simulink library "pmm"  (R2021b)
settings: Solver=VariableStepAuto  StartTime=0.0  StopTime=10.0  RelTol=1e-3
undefined symbols (not defined in the file or in its folder): APMM_CoolgFanActCurr_X_pct, APMM_EWP1Curr_X_c, APMM_EWP3Curr_X_c, APMM_LVBattChktime_X_enum, APMM_LVBattChrgtime_X_enum, APMM_LVChrgLv_X_mV, ENUM_ANTITHEFT_ALARM, ENUM_ANTITHEFT_ARM, ENUM_ANTITHEFT_DISARM, ENUM_ANTITHEFT_WAIT, ENUM_CHRGPLUGSTA_NONE, ENUM_CRASHSTATE_NOCRASH, ENUM_DCDCFAULTSTA_ANYFAULTLV1, ENUM_DCDCFAULTSTA_ANYFAULTLV2, ENUM_DRIVETRAIN_AWD, ENUM_DRIVETRAIN_FWD, ENUM_DRIVETRAIN_RWD, ENUM_GEARACTUALPOSN_D, ENUM_GEARACTUALPOSN_N, ENUM_GEARACTUALPOSN_R, ENUM_HVBATTREADYPRE_READY, ENUM_OTACHKSTA_NOREQUEST, ENUM_OTACHKSTA_NOTIMEOUT, ENUM_OTACHKSTA_TIMEOUT, ENUM_PDKEYRAWLULOCK_INLOCK, ENUM_PDKEYRAWLULOCK_INUNLOCK, ENUM_PDKEYRAWPS_INPS, ENUM_PDKEYSTA_LOCK, ENUM_PDKEYSTA_PS, ENUM_PDKEYSTA_UNAVALIABLE, ENUM_PDKEYSTA_UNLOCK, ENUM_POWERSTA_OFF, ENUM_POWERSTA_OFFC, ENUM_POWERSTA_STANDBY, ENUM_PWRREQOTA_REQPOWEROFF, ENUM_PWRREQOTA_REQPOWERSTDBY, ENUM_PWRSTASW_READY, FALSE, KPMM_AllDoorClosedHoldTime_s, KPMM_APSAllowThd_pct, KPMM_BattDownFailtime_s, KPMM_BattUpFailtime_s, KPMM_BattUpResetRty_cnt, KPMM_BattUpResetSW_flg, KPMM_BattUpResetTO_s, KPMM_BattUpRstDlyTO_s, KPMM_BrakeSWHoldTime_s, KPMM_ChrgPlugHoldTime_s, KPMM_DCDCDisableFailtime_s, KPMM_DCDCEnableFailtime_s, KPMM_DCDCVSET_V, KPMM_DCDCVSETLVChrg_V, KPMM_DoorSWHoldTime_s, KPMM_DriverSafetyChkFailtime_s, KPMM_DrivetrainSelect_enum_ovrdflg, KPMM_DrivetrainSelect_enum_ovrdval, KPMM_FDADC12VDetAccu_s, KPMM_FDADC12VDetAccuIntval_s, KPMM_FirstLVCheckHoldT_s, KPMM_FrMCUDischrgVolt_V ... (+54)
libraries: simulink x28, hcu_lib x13
(part 3 of 5)

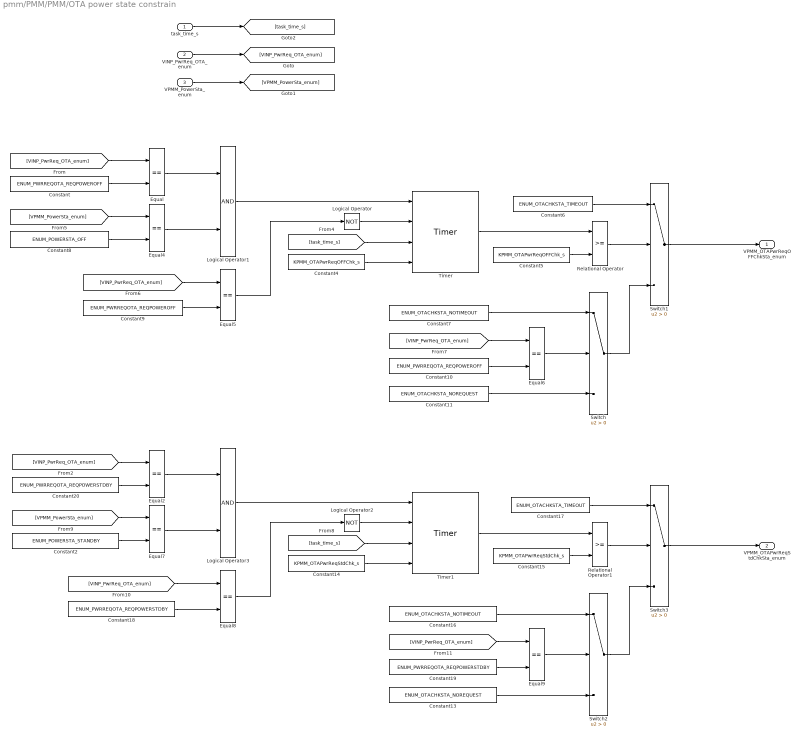
== system pmm/PMM/PMM/OTA power state constrain ==
  task_time_s : Inport
  VINP_PwrReq_OTA_enum : Inport  Port=2
  VPMM_PowerSta_enum : Inport  Port=3
  Constant : Constant  Value=ENUM_PWRREQOTA_REQPOWEROFF
  Constant10 : Constant  Value=ENUM_PWRREQOTA_REQPOWEROFF
  Constant11 : Constant  Value=ENUM_OTACHKSTA_NOREQUEST
  Constant13 : Constant  Value=ENUM_OTACHKSTA_NOREQUEST
  Constant14 : Constant  Value=KPMM_OTAPwrReqStdChk_s
  Constant15 : Constant  Value=KPMM_OTAPwrReqStdChk_s
  Constant16 : Constant  Value=ENUM_OTACHKSTA_NOTIMEOUT
  Constant17 : Constant  Value=ENUM_OTACHKSTA_TIMEOUT
  Constant18 : Constant  Value=ENUM_PWRREQOTA_REQPOWERSTDBY
  Constant19 : Constant  Value=ENUM_PWRREQOTA_REQPOWERSTDBY
  Constant2 : Constant  Value=ENUM_POWERSTA_STANDBY
  Constant20 : Constant  Value=ENUM_PWRREQOTA_REQPOWERSTDBY
  Constant4 : Constant  Value=KPMM_OTAPwrReqOFFChk_s
  Constant5 : Constant  Value=KPMM_OTAPwrReqOFFChk_s
  Constant6 : Constant  Value=ENUM_OTACHKSTA_TIMEOUT
  Constant7 : Constant  Value=ENUM_OTACHKSTA_NOTIMEOUT
  Constant8 : Constant  Value=ENUM_POWERSTA_OFF
  Constant9 : Constant  Value=ENUM_PWRREQOTA_REQPOWEROFF
  Equal{,2,4..9} (8 alike) : RelationalOperator  Operator===  OutDataTypeStr=boolean  RndMeth=Simplest
  Logical Operator : Logic  Operator=NOT  AllPortsSameDT=off  OutDataTypeStr=boolean
  Logical Operator1 : Logic  AllPortsSameDT=off  OutDataTypeStr=boolean
  Logical Operator2 : Logic  Operator=NOT  AllPortsSameDT=off  OutDataTypeStr=boolean
  Logical Operator3 : Logic  AllPortsSameDT=off  OutDataTypeStr=boolean
  Relational Operator : RelationalOperator  OutDataTypeStr=boolean  RndMeth=Simplest
  Relational Operator1 : RelationalOperator  OutDataTypeStr=boolean  RndMeth=Simplest
  Switch{,1..3} (4 alike) : Switch  Criteria=u2 > Threshold
  Timer : hcu_lib/Basic_Blocks/Timer
  Timer1 : hcu_lib/Basic_Blocks/Timer
  VPMM_OTAPwrReqOFFChkSta_enum : Outport
  VPMM_OTAPwrReqStdChkSta_enum : Outport  Port=2
  wires:
  Constant/1 -> Equal/2
  VINP_PwrReq_OTA_enum/1 -> [VINP_PwrReq_OTA_enum]
  VPMM_PowerSta_enum/1 -> [VPMM_PowerSta_enum]
  [VINP_PwrReq_OTA_enum] -> Equal/1
  task_time_s/1 -> [task_time_s]
  [task_time_s] -> Timer/3
  Constant4/1 -> Timer/4
  Constant5/1 -> Relational Operator/2
  Timer/1 -> Relational Operator/1
  Relational Operator/1 -> Switch1/2
  Logical Operator/1 -> Timer/2
  Constant8/1 -> Equal4/2
  [VPMM_PowerSta_enum] -> Equal4/1
  Equal/1 -> Logical Operator1/1
  Equal4/1 -> Logical Operator1/2
  Logical Operator1/1 -> Timer/1
  [VINP_PwrReq_OTA_enum] -> Equal5/1
  Constant9/1 -> Equal5/2
  Equal5/1 -> Logical Operator/1
  Constant6/1 -> Switch1/1
  Constant10/1 -> Equal6/2
  [VINP_PwrReq_OTA_enum] -> Equal6/1
  Equal6/1 -> Switch/2
  Constant7/1 -> Switch/1
  Switch/1 -> Switch1/3
  Constant11/1 -> Switch/3
  Switch1/1 -> VPMM_OTAPwrReqOFFChkSta_enum/1
  Switch2/1 -> Switch3/3
  Equal9/1 -> Switch2/2
  [VINP_PwrReq_OTA_enum] -> Equal9/1
  Equal8/1 -> Logical Operator2/1
  [VINP_PwrReq_OTA_enum] -> Equal8/1
  Logical Operator3/1 -> Timer1/1
  Equal7/1 -> Logical Operator3/2
  Equal2/1 -> Logical Operator3/1
  [VPMM_PowerSta_enum] -> Equal7/1
  Logical Operator2/1 -> Timer1/2
  Relational Operator1/1 -> Switch3/2
  Timer1/1 -> Relational Operator1/1
  Constant15/1 -> Relational Operator1/2
  Constant14/1 -> Timer1/4
  [task_time_s] -> Timer1/3
  [VINP_PwrReq_OTA_enum] -> Equal2/1
  Constant20/1 -> Equal2/2
  Constant13/1 -> Switch2/3
  Constant16/1 -> Switch2/1
  Constant17/1 -> Switch3/1
  Switch3/1 -> VPMM_OTAPwrReqStdChkSta_enum/1
  Constant2/1 -> Equal7/2
  Constant18/1 -> Equal8/2
  Constant19/1 -> Equal9/2

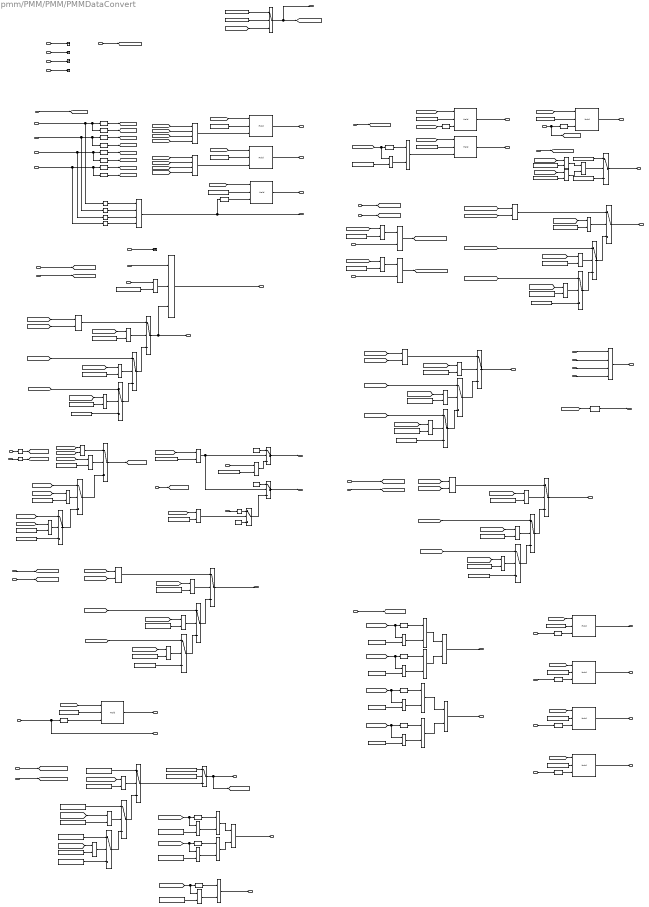
== system pmm/PMM/PMM/PMMDataConvert ==
  note: Detect HV power state
  note: Detect PW Continue Use
  note: Detect SchedChgwake
  note: Detect IVI Power OFF
  note: Monitor for DCDC fault level
  note: VPMM_SafetyChkMLv_flg
      | 0 Fail
      | 1 OK
  note: Safety Check
  note: VPMM_TMSpdThdSta_flg
      | 0 = Not allow MCU disable
      | 1 = Allow MCU disable
  note: 0 = HVIL close; 1 = HVIL open
  note: Seat Switch Rising Edge
  note: Detect Gun Plug Rising/Faling Edge
  note: KEY STATE
  note: Brake signal convert to rising edge
  note: Door judgement
  note: Precharge Check
  note: MCU Enable
  note: MCU Discharge
  note: MCU Ready
  note: Antitheft State
  note: OPDS Signal tramsmit function
  note: BMSWarn judgement
  note: MCU DC Bus Max Voltage judgement
  task_time_s : Inport
  VBCM_AntitheftSta_enum : Inport  Port=2
  VINP_DrDoorSW_flg : Inport  Port=3
  VINP_PsDoorSW_flg : Inport  Port=4
  VINP_RRDoorSW_flg : Inport  Port=5
  VINP_RLDoorSW_flg : Inport  Port=6
  VINP_BrakeSWGPIO_flg : Inport  Port=7
  VINP_FrMCUDCBusVolt_V : Inport  Port=8
  VINP_FrMCUDischrgSta_flg : Inport  Port=9
  VINP_FrMCUEnaSta_flg : Inport  Port=10
  VINP_FrMCUErr_enum : Inport  Port=11
  VINP_FrMCUReady4Pre_flg : Inport  Port=12
  VINP_FrMCUReady_flg : Inport  Port=13
  VINP_FrMCUTemp_C : Inport  Port=14
  VINP_RrMCUDCBusVolt_V : Inport  Port=15
  VINP_RrMCUDischrgSta_flg : Inport  Port=16
  VINP_RrMCUEnaSta_flg : Inport  Port=17
  VINP_RrMCUErr_enum : Inport  Port=18
  VINP_RrMCUReady4Pre_flg : Inport  Port=19
  VINP_RrMCUReady_flg : Inport  Port=20
  VINP_RrMCUTemp_C : Inport  Port=21
  VINP_DCDCReady4Pre_flg : Inport  Port=22
  VINP_OBCReady4Pre_flg : Inport  Port=23
  VINP_HVBattReady4Pre_enum : Inport  Port=24
  VINP_PDKeyAreaPS_enum : Inport  Port=25
  VINP_PDKeyAreaLockUnlock_enum : Inport  Port=26
  VINP_ChrgPlugSta_enum : Inport  Port=27
  VINP_SeatSW_flg : Inport  Port=28
  VINP_HVILSta_flg : Inport  Port=29
  VINP_CrashOutputSts_enum : Inport  Port=30
  VPMM_PowerSta_enum : Inport  Port=31
  VINP_RrTMSpd_rpm : Inport  Port=32
  VINP_FrTMSpd_rpm : Inport  Port=33
  VINP_BMSWarn5_flg : Inport  Port=34
  VINP_BMSWarn6_flg : Inport  Port=35
  VINP_BMSWarn7_flg : Inport  Port=36
  VINP_BMSWarn8_flg : Inport  Port=37
  VINP_DrivetrainSelect_enum : Inport  Port=38
  VINP_DCDCFaultSta_enum : Inport  Port=39
  VINP_IVIPwroffreq_flg : Inport  Port=40
  VINP_SchedChgwake_flg : Inport  Port=41
  VINP_PWCONTINUEUSE_flg : Inport  Port=42
  VPMM_HVPwrSta_flg : Inport  Port=43
  AND{,3..6,8} (6 alike) : Logic  AllPortsSameDT=off  OutDataTypeStr=boolean
  AND1 : Logic  Inputs=3  AllPortsSameDT=off  OutDataTypeStr=boolean
  AND7 : Logic  Operator=OR  Inputs=4  AllPortsSameDT=off  OutDataTypeStr=boolean
  Abs : Abs
  Abs1 : Abs
  Constant : Constant  Value=KPMM_DoorSWHoldTime_s
  Constant1 : Constant  Value=KPMM_DoorSWHoldTime_s
  Constant10 : Constant  Value=KPMM_TMSpdMCUDisThrsh_rpm
  Constant{4,11,19,22,30,38} (6 alike) : Constant  Value=ENUM_DRIVETRAIN_AWD
  Constant{12,29,33,36} (4 alike) : Constant  Value=TRUE
  Constant{6,13,21,32,39,46} (6 alike) : Constant  Value=ENUM_DRIVETRAIN_FWD
  Constant14 : Constant  Value=ENUM_HVBATTREADYPRE_READY
  Constant{8,15,23,34,40,51} (6 alike) : Constant  Value=ENUM_DRIVETRAIN_RWD
  Constant{7,9,16..17,28,35} (6 alike) : Constant  Value=FALSE
  Constant18 : Constant  Value=KPMM_ChrgPlugHoldTime_s
  Constant2 : Constant  Value=ZERO_FLOAT
  Constant20 : Constant  Value=KPMM_ChrgPlugHoldTime_s
  Constant24 : Constant  Value=KPMM_RrMCUDischrgVolt_V
  Constant25 : Constant  Value=KPMM_FrMCUDischrgVolt_V
  Constant26 : Constant  Value=KPMM_DrivetrainSelect_enum_ovrdflg
  Constant27 : Constant  Value=ENUM_POWERSTA_OFF
  Constant3 : Constant  Value=KPMM_SeatSWHoldTime_s
  Constant31 : Constant  Value=ENUM_CHRGPLUGSTA_NONE
  Constant37 : Constant  Value=KPMM_AllDoorClosedHoldTime_s
  Constant41 : Constant  Value=KPMM_BrakeSWHoldTime_s
  Constant42 : Constant  Value=KPMM_PDKeySta_enum_ovrdval
  Constant43 : Constant  Value=ENUM_PDKEYRAWPS_INPS
  Constant44 : Constant  Value=KPMM_PDKeySta_enum_ovrdflg
  Constant45 : Constant  Value=ENUM_PDKEYRAWLULOCK_INUNLOCK
  Constant47 : Constant  Value=ENUM_PDKEYRAWLULOCK_INLOCK
  Constant48 : Constant  Value=ENUM_PDKEYSTA_UNAVALIABLE
  Constant49 : Constant  Value=ENUM_PDKEYSTA_LOCK
  Constant5 : Constant  Value=ENUM_CRASHSTATE_NOCRASH
  Constant50 : Constant  Value=ENUM_PDKEYSTA_UNLOCK
  Constant52 : Constant  Value=KPMM_DrivetrainSelect_enum_ovrdval
  Constant53 : Constant  Value=ENUM_ANTITHEFT_DISARM
  Constant54 : Constant  Value=ENUM_ANTITHEFT_WAIT
  Constant55 : Constant  Value=ENUM_DCDCFAULTSTA_ANYFAULTLV1
  Constant56 : Constant  Value=ENUM_PDKEYSTA_PS
  Constant57 : Constant  Value=ENUM_DCDCFAULTSTA_ANYFAULTLV2
  Constant58 : Constant  Value=ENUM_PDKEYSTA_UNLOCK
  Constant59 : Constant  Value=ENUM_PDKEYSTA_PS
  Constant60 : Constant  Value=ENUM_ANTITHEFT_ARM
  Constant61 : Constant  Value=ENUM_ANTITHEFT_ALARM
  Constant62 : Constant  Value=ENUM_PDKEYSTA_LOCK
  Constant63 : Constant  Value=KPMM_IVIPwroffHoldTime_s
  Constant64 : Constant  Value=KPMM_SchedChgHoldTime_s
  Constant65 : Constant  Value=KPMM_PWCONTINUEHoldTime_s
  Constant66 : Constant  Value=KPMM_HVPwrStaHoldTime_s
  Data Type Conversion : DataTypeConversion  OutDataTypeStr=uint8
  Detect Change{,1..6} (7 alike) : simulink/Logic and Bit Operations/Detect Change  vinit=0  OutDataTypeStr=boolean
  Detect Decrease{,1..4} (5 alike) : simulink/Logic and Bit Operations/Detect Decrease  vinit=0.0  OutDataTypeStr=boolean
  Detect Increase{,1..11} (12 alike) : simulink/Logic and Bit Operations/Detect Increase  vinit=0.0  OutDataTypeStr=boolean
  Equal{,1..9,12..25,27..36} (34 alike) : RelationalOperator  Operator===  OutDataTypeStr=boolean  RndMeth=Simplest
  Equal10 : RelationalOperator  Operator=<=  OutDataTypeStr=boolean  RndMeth=Simplest
  Equal11 : RelationalOperator  Operator=<=  OutDataTypeStr=boolean  RndMeth=Simplest
  Equal26 : RelationalOperator  Operator=<  OutDataTypeStr=boolean  RndMeth=Simplest
  Hold{,1..10} (11 alike) : hcu_lib/Basic_Blocks/Hold  SystemSampleTime=-1  VariantActivationTime=update diagram  Latency=0  AutoFrameSizeCalculation=off
      settings: SourceProductName=HCU Relative Block Library
  LiuzgSwitch{1..15,18..26} (24 alike) : Switch  Criteria=u2 ~= 0
      settings: AttributesFormatString=<%<Criteria>>
  Logical Operator{,4,7,10} (4 alike) : Logic  Operator=OR  AllPortsSameDT=off  OutDataTypeStr=boolean
  Logical Operator{1..3,5..6,8..9,11} (8 alike) : Logic  AllPortsSameDT=off  OutDataTypeStr=boolean
  Max : MinMax  Function=max  Inputs=2
  Max1 : MinMax  Function=max  Inputs=2
  NOT{1..5} (5 alike) : Logic  Operator=NOT  AllPortsSameDT=off  OutDataTypeStr=boolean
  OR : Logic  Operator=OR  Inputs=4  AllPortsSameDT=off  OutDataTypeStr=boolean
  OR1 : Logic  Operator=OR  Inputs=4  AllPortsSameDT=off  OutDataTypeStr=boolean
  OR2 : Logic  Inputs=4  AllPortsSameDT=off  OutDataTypeStr=boolean
  Switch : Switch  Criteria=u2 ~= 0
  Switch1 : Switch  Criteria=u2 ~= 0
  Switch2 : Switch  Criteria=u2 > Threshold
  Terminator{,1..3,5} (5 alike) : Terminator
  VPMM_DetectDoorOpened_flg : Outport
  VPMM_DetectDoorClosed_flg : Outport  Port=2
  VPMM_BrkPedalPressed_flg : Outport  Port=3
  VPMM_PreChrgChk_flg : Outport  Port=4
  VPMM_AllDoorClosed_flg : Outport  Port=5
  VPMM_MCUEnable_flg : Outport  Port=6
  VPMM_MCUDischrgFinished_flg : Outport  Port=7
  VPMM_MCUReady_flg : Outport  Port=8
  VPMM_PDKeySta_enum : Outport  Port=9
  VPMM_BrkPedalRisingEdge_flg : Outport  Port=10
  VPMM_AllDoorCloseRisingEdge_flg : Outport  Port=11
  VPMM_DrivetrainSelect_enum : Outport  Port=12
  VPMM_ChrgPlugInRisingEdge_flg : Outport  Port=13
  VPMM_ChrgPlugOutFallingEdge_flg : Outport  Port=14
  VPMM_SeatSWRisingEdge_flg : Outport  Port=15
  VPMM_SafetyChkMLv_flg : Outport  Port=16
  VPMM_SafetyChkHLv_flg : Outport  Port=17
  VPMM_DrSeatSta_enum : Outport  Port=18
  VPMM_BMSWarm_flg : Outport  Port=19
  VPMM_MCUDCBusMaxVolt_V : Outport  Port=20
  VPMM_DetectAntitheftUnlock_flg : Outport  Port=21
  VPMM_LVSysErrPwrOutErr_flg : Outport  Port=22
  VPMM_DetectPDKeyUnlock_flg : Outport  Port=23
  VPMM_DetectAntitheftLock_flg : Outport  Port=24
  VPMM_DetectPDKeyLock_flg : Outport  Port=25
  VPMM_DetectIVIPwroffreq_flg : Outport  Port=26
  VPMM_DetectSchedChg_flg : Outport  Port=27
  VPMM_DetectPWCONTINUE_flg : Outport  Port=28
  VPMM_DetectHVPwrSta_flg : Outport  Port=29
  VPMM_MCUReady4Pre_flg : Outport  Port=30
  wires:
  [VPMM_PowerSta_enum] -> Equal13/1
  Data Type Conversion/1 -> VPMM_DrSeatSta_enum/1  "VPMM_DrSeatSta_enum"
  [VPMM_FrMCUDCBusVolt_V] -> Max1/2
  [VPMM_RrMCUDCBusVolt_V] -> Max1/1
  [VPMM_FrMCUDCBusVolt_V] -> LiuzgSwitch18/1
  Max1/1 -> LiuzgSwitch25/1
  Constant7/1 -> LiuzgSwitch26/3
  Constant46/1 -> Equal30/2
  LiuzgSwitch26/1 -> LiuzgSwitch18/3
  Equal12/1 -> LiuzgSwitch25/2
  Constant51/1 -> Equal31/2
  [VPMM_DrivetrainSelect_enum] -> Equal12/1
  Equal30/1 -> LiuzgSwitch18/2
  Constant22/1 -> Equal12/2
  LiuzgSwitch18/1 -> LiuzgSwitch25/3
  [VPMM_DrivetrainSelect_enum] -> Equal30/1
  Equal31/1 -> LiuzgSwitch26/2
  [VPMM_DrivetrainSelect_enum] -> Equal31/1
  [VPMM_RrMCUDCBusVolt_V] -> LiuzgSwitch26/1
  LiuzgSwitch25/1 -> VPMM_MCUDCBusMaxVolt_V/1  "VPMM_MCUDCBusMaxVolt_V"
  [VPMM_FrMCUDCBusVolt_V] -> Equal11/1
  [VPMM_RrMCUDCBusVolt_V] -> Equal10/1
  VINP_BMSWarn5_flg/1 -> AND7/1
  VINP_BMSWarn6_flg/1 -> AND7/2
  VINP_BMSWarn7_flg/1 -> AND7/3
  VINP_BMSWarn8_flg/1 -> AND7/4
  AND7/1 -> VPMM_BMSWarm_flg/1  "VPMM_BMSWarm_flg"
  [VPMM_SeatSW_flg] -> Data Type Conversion/1
  Abs1/1 -> [VINP_FrTMSpdABS_rpm]
  Abs/1 -> [VINP_RrTMSpdABS_rpm]
  Constant33/1 -> LiuzgSwitch19/3
  NOT1/1 -> LiuzgSwitch19/1
  [VPMM_TMSpd_rpm] -> Equal26/1
  LiuzgSwitch23/1 -> [VPMM_TMSpd_rpm]  "VPMM_TMSpd_rpm"
  Constant2/1 -> LiuzgSwitch24/3
  Max/1 -> LiuzgSwitch23/1
  [VINP_FrTMSpdABS_rpm] -> Max/2
  [VINP_RrTMSpdABS_rpm] -> Max/1
  LiuzgSwitch22/1 -> LiuzgSwitch23/3
  LiuzgSwitch24/1 -> LiuzgSwitch22/3
  [VINP_FrTMSpdABS_rpm] -> LiuzgSwitch22/1
  [VINP_RrTMSpdABS_rpm] -> LiuzgSwitch24/1
  [VPMM_DrivetrainSelect_enum] -> Equal27/1
  Constant40/1 -> Equal29/2
  Constant38/1 -> Equal27/2
  Equal29/1 -> LiuzgSwitch24/2
  Equal27/1 -> LiuzgSwitch23/2
  Constant39/1 -> Equal28/2
  [VPMM_DrivetrainSelect_enum] -> Equal29/1
  Equal28/1 -> LiuzgSwitch22/2
  [VPMM_DrivetrainSelect_enum] -> Equal28/1
  VINP_FrTMSpd_rpm/1 -> Abs1/1
  VINP_RrTMSpd_rpm/1 -> Abs/1
  Constant10/1 -> Equal26/2
  Equal/1 -> LiuzgSwitch21/3
  LiuzgSwitch19/1 -> LiuzgSwitch20/3
  Equal13/1 -> LiuzgSwitch21/2, LiuzgSwitch20/2
  LiuzgSwitch20/1 -> VPMM_SafetyChkMLv_flg/1  "VPMM_SafetyChkMLv_flg"
  LiuzgSwitch21/1 -> VPMM_SafetyChkHLv_flg/1  "VPMM_SafetyChkHLv_flg"
  VPMM_PowerSta_enum/1 -> [VPMM_PowerSta_enum]
  Constant5/1 -> Equal/2
  Constant12/1 -> LiuzgSwitch21/1
  Constant29/1 -> LiuzgSwitch20/1
  Constant27/1 -> Equal13/2
  VINP_CrashOutputSts_enum/1 -> Equal/1
  VINP_HVILSta_flg/1 -> NOT1/1
  Equal26/1 -> LiuzgSwitch19/2  "VPMM_TMSpdThdSta_flg"
  [task_time_s] -> Hold4/1
  Hold4/1 -> VPMM_SeatSWRisingEdge_flg/1  "VPMM_SeatSWRisingEdge_flg"
  VINP_SeatSW_flg/1 -> Detect Increase6/1, [VPMM_SeatSW_flg]
  Constant3/1 -> Hold4/2
  Detect Increase6/1 -> Hold4/3
  Constant18/1 -> Hold6/2
  Hold5/1 -> VPMM_ChrgPlugOutFallingEdge_flg/1  "VPMM_ChrgPlugOutFallingEdge_flg"
  Detect Increase7/1 -> Hold6/3
  [VINP_ChrgPlugSta_enum] -> Detect Increase7/1
  [task_time_s] -> Hold5/1
  VINP_ChrgPlugSta_enum/1 -> [VINP_ChrgPlugSta_enum]
  Constant20/1 -> Hold5/2
  [task_time_s] -> Hold6/1
  Logical Operator1/1 -> Hold5/3
  Hold6/1 -> VPMM_ChrgPlugInRisingEdge_flg/1  "VPMM_ChrgPlugInRisingEdge_flg"
  Equal25/1 -> Logical Operator1/2
  [VINP_ChrgPlugSta_enum] -> Detect Decrease4/1, Equal25/1
  Constant31/1 -> Equal25/2
  Detect Decrease4/1 -> Logical Operator1/1
  Equal24/1 -> AND1/2
  Constant14/1 -> Equal24/2
  Switch/1 -> VPMM_DrivetrainSelect_enum/1, [VPMM_DrivetrainSelect_enum]  "VPMM_DrivetrainSelect_enum"
  Detect Increase5/1 -> Hold2/3
  Hold2/1 -> VPMM_AllDoorCloseRisingEdge_flg/1  "VPMM_AllDoorCloseRisingEdge_flg"
  Constant37/1 -> Hold2/2
  [task_time_s] -> Hold2/1
  VINP_OBCReady4Pre_flg/1 -> Terminator1/1
  VINP_HVBattReady4Pre_enum/1 -> Equal24/1
  LiuzgSwitch14/1 -> Switch1/3
  Constant42/1 -> Switch1/1
  Switch1/1 -> [VPMM_PDKeySta_enum], VPMM_PDKeySta_enum/1  "VPMM_PDKeySta_enum"
  Constant44/1 -> Switch1/2
  Constant50/1 -> LiuzgSwitch13/1
  Constant56/1 -> LiuzgSwitch14/1
  Constant49/1 -> LiuzgSwitch15/1
  [VINP_PDKeyAreaLockUnlock_enum] -> Equal22/1
  Equal22/1 -> LiuzgSwitch15/2
  [VINP_PDKeyAreaLockUnlock_enum] -> Equal21/1
  LiuzgSwitch13/1 -> LiuzgSwitch14/3
  Constant43/1 -> Equal20/2
  Equal21/1 -> LiuzgSwitch13/2
  [VINP_PDKeyAreaPS_enum] -> Equal20/1
  Constant47/1 -> Equal22/2
  Equal20/1 -> LiuzgSwitch14/2
  LiuzgSwitch15/1 -> LiuzgSwitch13/3
  Constant45/1 -> Equal21/2
  Constant48/1 -> LiuzgSwitch15/3
  VINP_PDKeyAreaPS_enum/1 -> [VINP_PDKeyAreaPS_enum]
  Hold3/1 -> VPMM_BrkPedalRisingEdge_flg/1  "VPMM_BrkPedalRisingEdge_flg"
  [task_time_s] -> Hold3/1
  Constant41/1 -> Hold3/2
  Detect Increase4/1 -> Hold3/3  "VPMM_BrakePaddleRisingEdge_flg"
  [VPMM_DrivetrainSelect_enum] -> Equal15/1
  LiuzgSwitch10/1 -> LiuzgSwitch11/3
  LiuzgSwitch11/1 -> VPMM_MCUReady_flg/1  "VPMM_MCUReady_flg"
  [VINP_RrMCUReady_flg] -> LiuzgSwitch12/1
  Constant30/1 -> Equal14/2
  Constant28/1 -> LiuzgSwitch12/3
  Equal16/1 -> LiuzgSwitch12/2
  [VPMM_DrivetrainSelect_enum] -> Equal16/1
  AND8/1 -> LiuzgSwitch11/1
  [VINP_FrMCUReady_flg] -> AND8/1
  [VPMM_DrivetrainSelect_enum] -> Equal14/1
  Constant34/1 -> Equal16/2
  LiuzgSwitch12/1 -> LiuzgSwitch10/3
  VINP_RrMCUReady_flg/1 -> [VINP_RrMCUReady_flg]
  Constant32/1 -> Equal15/2
  [VINP_FrMCUReady_flg] -> LiuzgSwitch10/1
  VINP_FrMCUReady_flg/1 -> [VINP_FrMCUReady_flg]
  [VINP_RrMCUReady_flg] -> AND8/2
  Equal14/1 -> LiuzgSwitch11/2
  Equal15/1 -> LiuzgSwitch10/2
  VINP_RrMCUTemp_C/1 -> Terminator5/1
  VINP_RrMCUErr_enum/1 -> Terminator3/1
  VINP_FrMCUTemp_C/1 -> Terminator2/1
  VINP_FrMCUErr_enum/1 -> Terminator/1
  LiuzgSwitch8/1 -> VPMM_MCUDischrgFinished_flg/1  "VPMM_MCUDischrgFinished_flg"
  [VINP_RrDischrgComplete_flg] -> AND4/2
  [VINP_FrDischrgComplete_flg] -> AND4/1
  AND6/1 -> [VINP_FrDischrgComplete_flg]
  AND5/1 -> [VINP_RrDischrgComplete_flg]
  VINP_FrMCUDCBusVolt_V/1 -> [VPMM_FrMCUDCBusVolt_V]
  Constant25/1 -> Equal11/2
  Equal11/1 -> AND6/1
  VINP_FrMCUDischrgSta_flg/1 -> AND6/2
  VINP_RrMCUDischrgSta_flg/1 -> AND5/2
  Equal10/1 -> AND5/1
  Constant24/1 -> Equal10/2
  VINP_RrMCUDCBusVolt_V/1 -> [VPMM_RrMCUDCBusVolt_V]
  [VINP_RrDischrgComplete_flg] -> LiuzgSwitch9/1
  [VPMM_DrivetrainSelect_enum] -> Equal9/1
  Equal9/1 -> LiuzgSwitch9/2
  [VPMM_DrivetrainSelect_enum] -> Equal8/1
  LiuzgSwitch7/1 -> LiuzgSwitch8/3
  Constant19/1 -> Equal4/2
  Equal8/1 -> LiuzgSwitch7/2
  [VPMM_DrivetrainSelect_enum] -> Equal4/1
  Constant23/1 -> Equal9/2
  Equal4/1 -> LiuzgSwitch8/2
  LiuzgSwitch9/1 -> LiuzgSwitch7/3
  Constant21/1 -> Equal8/2
  Constant17/1 -> LiuzgSwitch9/3
  AND4/1 -> LiuzgSwitch8/1
  [VINP_FrDischrgComplete_flg] -> LiuzgSwitch7/1
  [VINP_RrMCUEnaSta_flg] -> AND3/2
  [VINP_FrMCUEnaSta_flg] -> AND3/1
  VINP_RrMCUEnaSta_flg/1 -> [VINP_RrMCUEnaSta_flg]
  VINP_FrMCUEnaSta_flg/1 -> [VINP_FrMCUEnaSta_flg]
  [VINP_FrMCUEnaSta_flg] -> LiuzgSwitch1/1
  AND3/1 -> LiuzgSwitch2/1
  Constant16/1 -> LiuzgSwitch3/3
  Constant6/1 -> Equal2/2
  LiuzgSwitch3/1 -> LiuzgSwitch1/3
  Equal1/1 -> LiuzgSwitch2/2
  Constant8/1 -> Equal3/2
  [VPMM_DrivetrainSelect_enum] -> Equal1/1
  Equal2/1 -> LiuzgSwitch1/2
  Constant4/1 -> Equal1/2
  LiuzgSwitch2/1 -> VPMM_MCUEnable_flg/1  "VPMM_MCUEnable_flg"
  LiuzgSwitch1/1 -> LiuzgSwitch2/3
  [VPMM_DrivetrainSelect_enum] -> Equal2/1
  Equal3/1 -> LiuzgSwitch3/2
  [VPMM_DrivetrainSelect_enum] -> Equal3/1
  [VINP_RrMCUEnaSta_flg] -> LiuzgSwitch3/1
  OR2/1 -> VPMM_AllDoorClosed_flg/1, Detect Increase5/1  "VPMM_AllDoorClosed_flg"
  NOT5/1 -> OR2/4
  NOT4/1 -> OR2/3
  NOT3/1 -> OR2/2
  NOT2/1 -> OR2/1
  AND1/1 -> VPMM_PreChrgChk_flg/1  "VPMM_PreChrgChk_flg"
  VINP_DCDCReady4Pre_flg/1 -> AND1/1
  LiuzgSwitch5/1 -> VPMM_MCUReady4Pre_flg/1, AND1/3  "VPMM_MCUReady4Pre_flg"
  [VINP_FrMCUReady4Pre_flg] -> AND/2
  [VINP_RrMCUReady4Pre_flg] -> AND/1
  VINP_FrMCUReady4Pre_flg/1 -> [VINP_FrMCUReady4Pre_flg]
  VINP_RrMCUReady4Pre_flg/1 -> [VINP_RrMCUReady4Pre_flg]
  [VINP_RrMCUReady4Pre_flg] -> LiuzgSwitch6/1
  [VPMM_DrivetrainSelect_enum] -> Equal6/1
  Equal6/1 -> LiuzgSwitch4/2
  [VINP_FrMCUReady4Pre_flg] -> LiuzgSwitch4/1
  Equal7/1 -> LiuzgSwitch6/2
  LiuzgSwitch4/1 -> LiuzgSwitch5/3
  [VPMM_DrivetrainSelect_enum] -> Equal7/1
  Constant11/1 -> Equal5/2
  Constant15/1 -> Equal7/2
  LiuzgSwitch6/1 -> LiuzgSwitch4/3
  AND/1 -> LiuzgSwitch5/1
  Constant13/1 -> Equal6/2
  Equal5/1 -> LiuzgSwitch5/2
  [VPMM_DrivetrainSelect_enum] -> Equal5/1
  Constant9/1 -> LiuzgSwitch6/3
  VINP_BrakeSWGPIO_flg/1 -> Detect Increase4/1, VPMM_BrkPedalPressed_flg/1
  [VPMM_FlClosed_flg] -> OR1/1
  [VPMM_FrClosed_flg] -> OR1/2
  [VPMM_RlClosed_flg] -> OR1/3
  [VPMM_RrClosed_flg] -> OR1/4
  Hold1/1 -> VPMM_DetectDoorClosed_flg/1  "VPMM_DetectDoorClosed_flg"
  OR1/1 -> Hold1/3
  [task_time_s] -> Hold1/1
  Constant1/1 -> Hold1/2
  Hold/1 -> VPMM_DetectDoorOpened_flg/1  "VPMM_DetectDoorOpened_flg"
  Constant/1 -> Hold/2
  [task_time_s] -> Hold/1
  OR/1 -> Hold/3
  task_time_s/1 -> [task_time_s]
  [VPMM_RrOpened_flg] -> OR/4
  [VPMM_RlOpened_flg] -> OR/3
  [VPMM_FlOpened_flg] -> OR/1
  [VPMM_FrOpened_flg] -> OR/2
  Detect Decrease3/1 -> [VPMM_RrClosed_flg]
  Detect Increase3/1 -> [VPMM_RrOpened_flg]
  Detect Decrease2/1 -> [VPMM_RlClosed_flg]
  Detect Increase2/1 -> [VPMM_RlOpened_flg]
  Detect Decrease1/1 -> [VPMM_FrClosed_flg]
  Detect Increase1/1 -> [VPMM_FrOpened_flg]
  Detect Decrease/1 -> [VPMM_FlClosed_flg]
  Detect Increase/1 -> [VPMM_FlOpened_flg]
  VINP_RLDoorSW_flg/1 -> Detect Increase3/1, Detect Decrease3/1, NOT5/1
  VINP_RRDoorSW_flg/1 -> Detect Increase2/1, Detect Decrease2/1, NOT4/1
  VINP_PsDoorSW_flg/1 -> Detect Increase1/1, Detect Decrease1/1, NOT3/1
  VINP_DrDoorSW_flg/1 -> Detect Increase/1, Detect Decrease/1, NOT2/1
  Constant26/1 -> Switch/2
  VINP_DrivetrainSelect_enum/1 -> [VINP_DrivetrainSelect_enum]
  [VINP_DrivetrainSelect_enum] -> Switch/3
  Constant52/1 -> Switch/1
  Detect Change1/1 -> Logical Operator3/1
  Logical Operator3/1 -> Logical Operator4/2
  Constant54/1 -> Equal17/2
  Logical Operator2/1 -> Logical Operator4/1
  Equal17/1 -> Logical Operator3/2
  Detect Change/1 -> Logical Operator2/1
  Logical Operator4/1 -> VPMM_DetectAntitheftUnlock_flg/1  "VPMM_DetectAntitheftUnlock_flg"
  [VBCM_AntitheftSta_enum] -> Detect Change/1, Equal18/1
  [VBCM_AntitheftSta_enum] -> Detect Change1/1, Equal17/1
  Equal18/1 -> Logical Operator2/2
  Constant53/1 -> Equal18/2
  VBCM_AntitheftSta_enum/1 -> [VBCM_AntitheftSta_enum]
  Switch2/1 -> VPMM_LVSysErrPwrOutErr_flg/1  "VPMM_LVSysErrPwrOutErr_flg"
  Constant35/1 -> Switch2/3
  Constant36/1 -> Switch2/1
  VINP_DCDCFaultSta_enum/1 -> [VINP_DCDCFaultSta_enum]
  [VINP_DCDCFaultSta_enum] -> Equal19/1
  [VINP_DCDCFaultSta_enum] -> Equal23/1
  Logical Operator/1 -> Switch2/2
  Equal19/1 -> Logical Operator/1
  Equal23/1 -> Logical Operator/2
  Constant55/1 -> Equal19/2
  Constant57/1 -> Equal23/2
  Constant59/1 -> Equal32/2
  Constant58/1 -> Equal33/2
  [VPMM_PDKeySta_enum] -> Equal32/1, Detect Change2/1
  [VPMM_PDKeySta_enum] -> Detect Change3/1, Equal33/1
  Detect Change2/1 -> Logical Operator5/1
  Equal32/1 -> Logical Operator5/2
  Detect Change3/1 -> Logical Operator6/1
  Equal33/1 -> Logical Operator6/2
  Logical Operator5/1 -> Logical Operator7/1
  Logical Operator6/1 -> Logical Operator7/2
  Logical Operator7/1 -> VPMM_DetectPDKeyUnlock_flg/1  "VPMM_DetectPDKeyUnlock_flg"
  [VBCM_AntitheftSta_enum] -> Equal34/1, Detect Change4/1
  Detect Change4/1 -> Logical Operator8/1
  Equal34/1 -> Logical Operator8/2
  Constant60/1 -> Equal34/2
  Constant61/1 -> Equal35/2
  Equal35/1 -> Logical Operator9/2
  Detect Change5/1 -> Logical Operator9/1
  [VBCM_AntitheftSta_enum] -> Detect Change5/1, Equal35/1
  Logical Operator8/1 -> Logical Operator10/1
  Logical Operator9/1 -> Logical Operator10/2
  Logical Operator10/1 -> VPMM_DetectAntitheftLock_flg/1  "VPMM_DetectAntitheftLock_flg"
  [VPMM_PDKeySta_enum] -> Detect Change6/1, Equal36/1
  Constant62/1 -> Equal36/2
  Detect Change6/1 -> Logical Operator11/1
  Equal36/1 -> Logical Operator11/2
  Logical Operator11/1 -> VPMM_DetectPDKeyLock_flg/1  "VPMM_DetectPDKeyLock_flg"
  [task_time_s] -> Hold7/1
  Constant63/1 -> Hold7/2
  Detect Increase8/1 -> Hold7/3
  VINP_IVIPwroffreq_flg/1 -> Detect Increase8/1
  Hold7/1 -> VPMM_DetectIVIPwroffreq_flg/1  "VPMM_DetectIVIPwroffreq_flg"
  Hold8/1 -> VPMM_DetectSchedChg_flg/1  "VPMM_DetectSchedChg_flg"
  Detect Increase9/1 -> Hold8/3
  VINP_SchedChgwake_flg/1 -> Detect Increase9/1
  Constant64/1 -> Hold8/2
  [task_time_s] -> Hold8/1
  [task_time_s] -> Hold9/1
  Constant65/1 -> Hold9/2
  Detect Increase10/1 -> Hold9/3
  VINP_PWCONTINUEUSE_flg/1 -> Detect Increase10/1
  Hold9/1 -> VPMM_DetectPWCONTINUE_flg/1  "VPMM_DetectPWCONTINUE_flg"
  VINP_PDKeyAreaLockUnlock_enum/1 -> [VINP_PDKeyAreaLockUnlock_enum]
  Detect Increase11/1 -> Hold10/3
  Constant66/1 -> Hold10/2
  [task_time_s] -> Hold10/1
  VPMM_HVPwrSta_flg/1 -> Detect Increase11/1
  Hold10/1 -> VPMM_DetectHVPwrSta_flg/1  "VPMM_DetectHVPwrSta_flg"

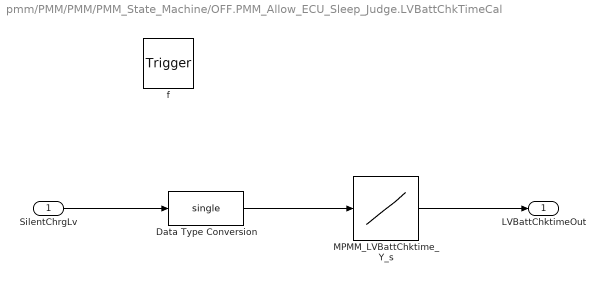
== system pmm/PMM/PMM/PMM_State_Machine/OFF.PMM_Allow_ECU_Sleep_Judge.LVBattChkTimeCal ==
  SilentChrgLv : Inport
  f : TriggerPort  TriggerType=function-call  VariantControl=(inherit)
      settings: CopyFcn=Stateflow.SLINSF.SimulinkMan.removeBlockPreDeleteFcn  PreDeleteFcn=Stateflow.SLINSF.SimulinkMan.unsafePredeleteFcn
  Data Type Conversion : DataTypeConversion  OutDataTypeStr=single
  MPMM_LVBattChktime_Y_s : Lookup_n-D  NumberOfTableDimensions=1  BreakpointsForDimension1=APMM_LVBattChktime_X_enum  Table=MPMM_LVBattChktime_Y_s  ExtrapMethod=Clip  InternalRulePriority=Speed  RndMeth=Simplest  InputSameDT=on
  LVBattChktimeOut : Outport
  wires:
  MPMM_LVBattChktime_Y_s/1 -> LVBattChktimeOut/1
  SilentChrgLv/1 -> Data Type Conversion/1
  Data Type Conversion/1 -> MPMM_LVBattChktime_Y_s/1

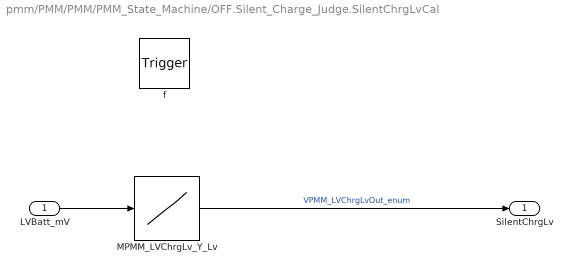
== system pmm/PMM/PMM/PMM_State_Machine/OFF.Silent_Charge_Judge.SilentChrgLvCal ==
  LVBatt_mV : Inport
  f : TriggerPort  TriggerType=function-call  VariantControl=(inherit)
      settings: CopyFcn=Stateflow.SLINSF.SimulinkMan.removeBlockPreDeleteFcn  PreDeleteFcn=Stateflow.SLINSF.SimulinkMan.unsafePredeleteFcn
  MPMM_LVChrgLv_Y_Lv : Lookup_n-D  NumberOfTableDimensions=1  BreakpointsForDimension1=APMM_LVChrgLv_X_mV  Table=MPMM_LVChrgLv_Y_Lv  ExtrapMethod=Clip  InternalRulePriority=Speed  RndMeth=Simplest  InputSameDT=on
  SilentChrgLv : Outport
  wires:
  LVBatt_mV/1 -> MPMM_LVChrgLv_Y_Lv/1
  MPMM_LVChrgLv_Y_Lv/1 -> SilentChrgLv/1  "VPMM_LVChrgLvOut_enum"

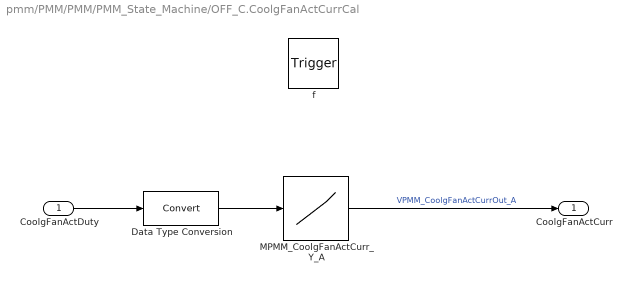
== system pmm/PMM/PMM/PMM_State_Machine/OFF_C.CoolgFanActCurrCal ==
  CoolgFanActDuty : Inport
  f : TriggerPort  TriggerType=function-call  VariantControl=(inherit)
      settings: CopyFcn=Stateflow.SLINSF.SimulinkMan.removeBlockPreDeleteFcn  PreDeleteFcn=Stateflow.SLINSF.SimulinkMan.unsafePredeleteFcn
  Data Type Conversion : DataTypeConversion
  MPMM_CoolgFanActCurr_Y_A : Lookup_n-D  NumberOfTableDimensions=1  BreakpointsForDimension1=APMM_CoolgFanActCurr_X_pct  Table=MPMM_CoolgFanActCurr_Y_A  ExtrapMethod=Clip  InternalRulePriority=Speed  RndMeth=Simplest  InputSameDT=on
  CoolgFanActCurr : Outport
  wires:
  MPMM_CoolgFanActCurr_Y_A/1 -> CoolgFanActCurr/1  "VPMM_CoolgFanActCurrOut_A"
  CoolgFanActDuty/1 -> Data Type Conversion/1
  Data Type Conversion/1 -> MPMM_CoolgFanActCurr_Y_A/1

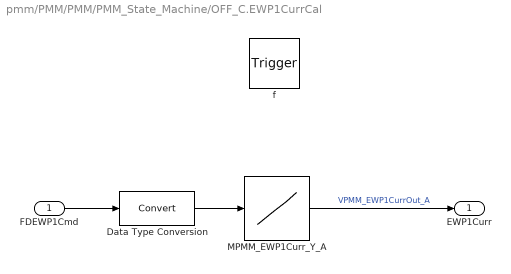
== system pmm/PMM/PMM/PMM_State_Machine/OFF_C.EWP1CurrCal ==
  FDEWP1Cmd : Inport
  f : TriggerPort  TriggerType=function-call  VariantControl=(inherit)
      settings: CopyFcn=Stateflow.SLINSF.SimulinkMan.removeBlockPreDeleteFcn  PreDeleteFcn=Stateflow.SLINSF.SimulinkMan.unsafePredeleteFcn
  Data Type Conversion : DataTypeConversion
  MPMM_EWP1Curr_Y_A : Lookup_n-D  NumberOfTableDimensions=1  BreakpointsForDimension1=APMM_EWP1Curr_X_c  Table=MPMM_EWP1Curr_Y_A  ExtrapMethod=Clip  InternalRulePriority=Speed  RndMeth=Simplest  InputSameDT=on
  EWP1Curr : Outport
  wires:
  MPMM_EWP1Curr_Y_A/1 -> EWP1Curr/1  "VPMM_EWP1CurrOut_A"
  FDEWP1Cmd/1 -> Data Type Conversion/1
  Data Type Conversion/1 -> MPMM_EWP1Curr_Y_A/1

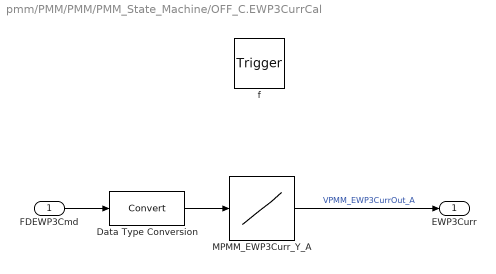
== system pmm/PMM/PMM/PMM_State_Machine/OFF_C.EWP3CurrCal ==
  FDEWP3Cmd : Inport
  f : TriggerPort  TriggerType=function-call  VariantControl=(inherit)
      settings: CopyFcn=Stateflow.SLINSF.SimulinkMan.removeBlockPreDeleteFcn  PreDeleteFcn=Stateflow.SLINSF.SimulinkMan.unsafePredeleteFcn
  Data Type Conversion : DataTypeConversion
  MPMM_EWP3Curr_Y_A : Lookup_n-D  NumberOfTableDimensions=1  BreakpointsForDimension1=APMM_EWP3Curr_X_c  Table=MPMM_EWP3Curr_Y_A  ExtrapMethod=Clip  InternalRulePriority=Speed  RndMeth=Simplest  InputSameDT=on
  EWP3Curr : Outport
  wires:
  MPMM_EWP3Curr_Y_A/1 -> EWP3Curr/1  "VPMM_EWP3CurrOut_A"
  FDEWP3Cmd/1 -> Data Type Conversion/1
  Data Type Conversion/1 -> MPMM_EWP3Curr_Y_A/1

== system pmm/PMM/PMM/PMM_State_Machine/OFF_C.LVBattChrgTimeCal ==
  SilentChrgLv : Inport
  f : TriggerPort  TriggerType=function-call  VariantControl=(inherit)
      settings: CopyFcn=Stateflow.SLINSF.SimulinkMan.removeBlockPreDeleteFcn  PreDeleteFcn=Stateflow.SLINSF.SimulinkMan.unsafePredeleteFcn
  MPMM_LVBattChrgtime_Y_s : Lookup_n-D  NumberOfTableDimensions=1  BreakpointsForDimension1=APMM_LVBattChrgtime_X_enum  Table=MPMM_LVBattChrgtime_Y_s  ExtrapMethod=Clip  InternalRulePriority=Speed  RndMeth=Simplest  InputSameDT=on
  LVBattChrgTime : Outport
  wires:
  MPMM_LVBattChrgtime_Y_s/1 -> LVBattChrgTime/1  "VPMM_LVBattChrgtimeOut_s"
  SilentChrgLv/1 -> MPMM_LVBattChrgtime_Y_s/1

== stateflow chart pmm/PMM/PMM/RequirementManagementForPowerUp ==
  state RequirementManagementForPowerUp
    (default) -> (junction 135)
    RequirementManagementForPowerUp -> (junction 135) [order 2]
    (junction 135) -> (junction 3) : {VPMM_PwrUpReq_enum = ENUM_PWRUPREQ_NOREQUEST;
        |  VPMM_PwrStaSelect_enum = ENUM_PWRSTASELECT_NOREQUEST;}
    (junction 3) -> (junction 158) [order 1] : [(VPMM_PowerSta_enum == ENUM_POWERSTA_OFF || ...
        |   VPMM_PowerSta_enum == ENUM_POWERSTA_STANDBY) && ...
        |  VPMM_OTAPwrReqOFFChkSta_enum != ENUM_OTACHKSTA_NOTIMEOUT && ...
        |  VPMM_OTAPwrReqStdChkSta_enum != ENUM_OTACHKSTA_NOTIMEOUT]
    (junction 158) -> (junction 5) [order 1] : [(VPMM_DetectDoorOpened_flg || ...
        |   VPMM_BrkPedalRisingEdge_flg || ...
        |   (VPMM_BrkPedalPressed_flg && VPMM_PreOFF_flg) || ...
        |   (VPMM_DetectDoorOpened_flg && VPMM_PreOFF_flg)) && ...
        |  VPMM_PowerSta_enum == ENUM_POWERSTA_STANDBY]
        | {VPMM_PwrStaSelect_enum = ENUM_PWRSTASELECT_GOON;}
    (junction 3) -> (junction 6) [order 2]
    (junction 158) -> (junction 7) [order 2]
    (junction 5) -> (junction 8)
    (junction 7) -> (junction 235) [order 1] : [VPMM_ChrgPlugInRisingEdge_flg && ...
        |  VPMM_PowerSta_enum == ENUM_POWERSTA_STANDBY]
        | {VPMM_PwrStaSelect_enum = ENUM_PWRSTASELECT_GOOFFC;}
    (junction 8) -> (junction 167) [order 1] : [VPMM_PowerUpState_enum == ENUM_PUSTATE_POWERUPFAIL]
    (junction 7) -> (junction 162) [order 2]
    (junction 235) -> (junction 173)
    (junction 8) -> (junction 169) [order 2] : {VPMM_PwrUpReq_enum = ENUM_PWRUPREQ_USERREQPU;}
    (junction 167) -> (junction 171)
    (junction 162) -> (junction 164) [order 1] : [VPMM_LVSilentChrgReqStd_flg || VPMM_LVSilentChrgReq_flg || ...
        |  (VINP_EvccAplusPwrUpReq_flg && VINP_ChrgPlugSta_enum != ENUM_CHRGPLUGSTA_NONE)]
        | {VPMM_PwrStaSelect_enum = ENUM_PWRSTASELECT_GOOFFC;}
    (junction 164) -> (junction 173) [order 1] : [VTQD_GearActualPosn_enum == ENUM_GEARACTUALPOSN_P && ...
        |  VINP_VehSpeed_kph < 2 && ...
        |  !VINP_HoodSW_flg]
    (junction 162) -> (junction 237) [order 2]
    (junction 164) -> (junction 225) [order 2]
    (junction 173) -> (junction 239)
    (junction 237) -> (junction 239) [order 1] : [VINP_PwrReq_OTA_enum == ENUM_PWRREQOTA_REQPOWERON && ...
        |  VINP_HVBattSOC_pct > KPMM_HVBattSOCPwrDwnThd_pct]
        | {VPMM_PwrStaSelect_enum = ENUM_PWRSTASELECT_GOON;}
    (junction 237) -> (junction 242) [order 2]
    (junction 239) -> (junction 244)
    (junction 242) -> (junction 244) [order 1] : [(VINP_SchedChgwake_flg == ENUM_SCHEDCHG_WAKE && ...
        |   VINP_ChrgPlugSta_enum == ENUM_CHRGPLUGSTA_AC)]
        | {VPMM_PwrStaSelect_enum = ENUM_PWRSTASELECT_GOOFFC;}
    (junction 242) -> (junction 248) [order 2]
    (junction 244) -> (junction 250)
    (junction 248) -> (junction 250) [order 1] : [VINP_HVBPreheatPrecoolSta_enum == ENUM_HVBPRESTA_PREHEAT || ...
        |  VINP_HVBPreheatPrecoolSta_enum == ENUM_HVBPRESTA_PRECOOL]
        | {VPMM_PwrStaSelect_enum = ENUM_PWRSTASELECT_GOOFFA;}
    (junction 248) -> (junction 179) [order 2]
    (junction 250) -> (junction 194)
    (junction 179) -> (junction 181) [order 1] : [VINP_RePwrReqTbox_enum == ENUM_REPWRREQTBOX_REQVEHCHK || ...
        |  VINP_RePwrReqTbox_enum == ENUM_REPWRREQTBOX_REQDTC || ...
        |  VINP_RePwrReqTbox_enum == ENUM_REPWRREQTBOX_REQRADIO || ...
        |  VINP_RePwrReqTbox_enum == ENUM_REPWRREQTBOX_REQON || ...
        |  VINP_RePwrReqDKCT_enum == ENUM_REPWRREQDKC_REQVEHCHK || ...
        |  VINP_RePwrReqDKCT_enum == ENUM_REPWRREQDKC_REQDTC || ...
        |  VINP_RePwrReqDKCT_enum == ENUM_REPWRREQDKC_REQRADIO || ...
        |  VINP_RePwrReqDKCT_enum == ENUM_REPWRREQDKC_REQON]
        | {VPMM_PwrStaSelect_enum = ENUM_PWRSTASELECT_GOON;}
    (junction 179) -> (junction 183) [order 2]
    (junction 181) -> (junction 185)
    (junction 183) -> (junction 185) [order 1] : [VINP_RePwrReqTbox_enum == ENUM_REPWRREQTBOX_REQACTEMP || ...
        |  VINP_RePwrReqDKCT_enum == ENUM_REPWRREQDKC_REQACTEMP]
        | {VPMM_PwrStaSelect_enum = ENUM_PWRSTASELECT_GOOFFA;}
    (junction 183) -> (junction 190) [order 2]
    (junction 185) -> (junction 9)
    (junction 9) -> (junction 194) [order 1] : [VTQD_GearActualPosn_enum == ENUM_GEARACTUALPOSN_P && ...
        |  !VPMM_BMSWarn_flg && ...
        |  VINP_VehSpeed_kph < 2 && ...
        |  VINP_HVBattSOC_pct > KPMM_HVBattSOCPwrDwnThd_pct && ...
        |  VPMM_AllDoorClosed_flg && ...
        |  !VINP_HoodSW_flg && ...
        |  !VINP_TailgateSW_flg && ...
        |  VBCM_AntitheftSta_enum == ENUM_ANTITHEFT_ARM]
        | {VPMM_ReVehThdChkSta_enum = ENUM_REVEHSTA_CHECKOK;}
    (junction 194) -> (junction 197) [order 1] : [VPMM_PowerUpState_enum == ENUM_PUSTATE_POWERUPFAIL]
    (junction 9) -> (junction 11) [order 2]
    (junction 194) -> (junction 204) [order 2] : {VPMM_PwrUpReq_enum = ENUM_PWRUPREQ_SYSREQPU;}
    (junction 197) -> (junction 200)
    (junction 11) -> (junction 12) [order 1] : [VTQD_GearActualPosn_enum != ENUM_GEARACTUALPOSN_P]
        | {VPMM_ReVehThdChkSta_enum = ENUM_REVEHSTA_GEARPOSITIONERROR;}
    (junction 11) -> (junction 15) [order 2]
    (junction 15) -> (junction 16) [order 1] : [VPMM_BMSWarn_flg]
        | {VPMM_ReVehThdChkSta_enum = ENUM_REVEHSTA_HVBERR;}
    (junction 15) -> (junction 17) [order 2]
    (junction 17) -> (junction 18) [order 1] : [VINP_VehSpeed_kph >= 2]
        | {VPMM_ReVehThdChkSta_enum = ENUM_REVEHSTA_VEHNOTSTEADYSTATE;}
    (junction 17) -> (junction 21) [order 2]
    (junction 21) -> (junction 22) [order 1] : [VBCM_AntitheftSta_enum != ENUM_ANTITHEFT_ARM]
        | {VPMM_ReVehThdChkSta_enum = ENUM_REVEHSTA_ANTITHEFTNOTARM;}
    (junction 21) -> (junction 26) [order 2]
    (junction 26) -> (junction 27) [order 1] : [!VPMM_AllDoorClosed_flg || ...
        |  VINP_HoodSW_flg || ...
        |  VINP_TailgateSW_flg]
        | {VPMM_ReVehThdChkSta_enum = ENUM_REVEHSTA_ANYDOOROPEN;}
    (junction 26) -> (junction 29) [order 2]
    (junction 29) -> (junction 30) [order 1] : [VINP_HVBattSOC_pct <= KPMM_HVBattSOCPwrDwnThd_pct]
        | {VPMM_ReVehThdChkSta_enum = ENUM_REVEHSTA_HVBSOCLOW;}
    (junction 29) -> (junction 31) [order 2] : {VPMM_ReVehThdChkSta_enum = ENUM_REVEHSTA_CHECKINVALID;}
    (junction 169) -> (junction 204)
    (junction 204) -> (junction 32)
    RequirementManagementForPowerUp -> (junction 32) [order 1] : [VPMM_PwrUpChk_flg]
        | {VPMM_PwrUpChk_flg = FALSE;}
    (junction 32) -> (junction 139) [order 1] : [VPMM_PowerUpState_enum == ENUM_PUSTATE_COMPLETED]
        | {VPMM_PwrUpChkFailtimer_s = 0;}
    (junction 32) -> (junction 141) [order 2]
    (junction 141) -> (junction 143) [order 1] : [VPMM_PwrUpChkFailtimer_s >= KPMM_PwrUpChkFailtime_s]
        | {VPMM_PwrUpChkFailtimer_s = 0;}
    (junction 141) -> (junction 145) [order 2] : {VPMM_PwrUpChk_flg = TRUE;
        |  VPMM_PwrUpChkFailtimer_s += task_time_s;}
  data: task_time_s input; VINP_HVBPreheatPrecoolSta_enum input; VINP_HVBattSOC_pct input; VINP_HoodSW_flg input; VINP_TailgateSW_flg input; VINP_SchedChgwake_flg input; VINP_VehSpeed_kph input; VPMM_AllDoorClosed_flg input; VBCM_AntitheftSta_enum input; VPMM_BMSWarn_flg input; VPMM_BrkPedalPressed_flg input; VPMM_BrkPedalRisingEdge_flg input; VPMM_ChrgPlugInRisingEdge_flg input; VPMM_DetectDoorOpened_flg input; VPMM_LVSilentChrgReq_flg input boolean; VPMM_PowerSta_enum input uint8; VTQD_GearActualPosn_enum input; VINP_PwrReq_OTA_enum input; VINP_RePwrReqDKCT_enum input; VINP_RePwrReqTbox_enum input; VPMM_PwrStaSelect_enum output; VPMM_PwrUpReq_enum output; VPMM_ReVehThdChkSta_enum output; ENUM_ANTITHEFT_ARM parameter; ENUM_GEARACTUALPOSN_P parameter; ENUM_HVBPRESTA_PRECOOL parameter; ENUM_HVBPRESTA_PREHEAT parameter; ENUM_POWERSTA_OFF parameter; ENUM_POWERSTA_STANDBY parameter; ENUM_PWRREQOTA_REQPOWERON parameter; ENUM_PWRSTASELECT_GOOFFA parameter; ENUM_PWRSTASELECT_GOOFFC parameter; ENUM_PWRSTASELECT_GOON parameter; ENUM_PWRSTASELECT_NOREQUEST parameter; ENUM_PWRUPREQ_NOREQUEST parameter; ENUM_PWRUPREQ_SYSREQPU parameter; ENUM_PWRUPREQ_USERREQPU parameter; ENUM_REPWRREQDKC_REQACTEMP parameter; ENUM_REPWRREQDKC_REQDTC parameter; ENUM_REPWRREQDKC_REQON parameter; ENUM_REPWRREQDKC_REQRADIO parameter; ENUM_REPWRREQDKC_REQVEHCHK parameter; ENUM_REPWRREQTBOX_REQACTEMP parameter; ENUM_REPWRREQTBOX_REQDTC parameter; ENUM_REPWRREQTBOX_REQON parameter; ENUM_REPWRREQTBOX_REQRADIO parameter; ENUM_REPWRREQTBOX_REQVEHCHK parameter; ENUM_REVEHSTA_ANTITHEFTNOTARM parameter; ENUM_REVEHSTA_ANYDOOROPEN parameter; ENUM_REVEHSTA_CHECKINVALID parameter; ENUM_REVEHSTA_CHECKOK parameter; ENUM_REVEHSTA_GEARPOSITIONERROR parameter; ENUM_REVEHSTA_HVBERR parameter; ENUM_REVEHSTA_HVBSOCLOW parameter; ENUM_REVEHSTA_VEHNOTSTEADYSTATE parameter; ENUM_SCHEDCHG_WAKE parameter; KPMM_PwrUpChkFailtime_s parameter; VPMM_PowerUpState_enum input uint8; VPMM_PwrUpChkFailtimer_s local single; VPMM_PwrUpChk_flg local boolean; ENUM_PUSTATE_COMPLETED parameter; FALSE parameter; TRUE parameter; VINP_ChrgPlugSta_enum input uint8; VINP_EvccAplusPwrUpReq_flg input boolean; VPMM_LVSilentChrgReqStd_flg input boolean; ENUM_CHRGPLUGSTA_AC parameter; ENUM_PUSTATE_POWERUPFAIL parameter; VPMM_PreOFF_flg input boolean; ENUM_CHRGPLUGSTA_NONE parameter; VPMM_OTAPwrReqOFFChkSta_enum input uint8; VPMM_OTAPwrReqStdChkSta_enum input uint8; ENUM_OTACHKSTA_NOTIMEOUT parameter; KPMM_HVBattSOCPwrDwnThd_pct input

== stateflow chart pmm/PMM/PMM/RequirementManagementForPowerStateConstrain ==
  state RequirementManagementForPowerStateConstrain
    (default) -> (junction 2) : {VPMM_TCountSta_enum = ENUM_TCOUNTSTA_NOCOUNTING;
        |  VPMM_PwrOffTimer_s = 0;}
    RequirementManagementForPowerStateConstrain -> (junction 2) [order 2]
    (junction 2) -> (junction 3) : {VPMM_PwrStaConstraint_enum = ENUM_PWRCONSTRAINT_NOREQUEST;}
    RequirementManagementForPowerStateConstrain -> (junction 3) [order 1] : [VPMM_ConstraintLoop_flg]
        | {VPMM_ConstraintLoop_flg = FALSE;}
    (junction 3) -> (junction 4) [order 1] : [VPMM_PowerSta_enum == ENUM_POWERSTA_ON || ...
        |  VPMM_PowerSta_enum == ENUM_POWERSTA_OFFA || ...
        |  VPMM_PowerSta_enum == ENUM_POWERSTA_OFFC]
    (junction 4) -> (junction 5) [order 1] : [VINP_PwrReq_OTA_enum == ENUM_PWRREQOTA_REQPOWERON || ...
        |  VINP_OFFACMODE_enum == ENUM_OFFACMODE_CAMP]
    (junction 3) -> (junction 6) [order 2]
    (junction 4) -> (junction 7) [order 2]
    (junction 5) -> (junction 8) : {VPMM_PwrStaConstraint_enum = ENUM_PWRCONSTRAINT_PWRSTAON;}
    (junction 7) -> (junction 8) [order 1] : [VINP_AVMOFFRecButt_flg == ENUM_AVMOFFRECBUTT_ON || ...
        |  VINP_OFFACMODE_enum == ENUM_OFFACMODE_PET || ...
        |  VINP_OFFACMODE_enum == ENUM_OFFACMODE_ON || ...
        |  VINP_HVBPreheatPrecoolSta_enum == ENUM_HVBPRESTA_PREHEAT || ...
        |  VINP_HVBPreheatPrecoolSta_enum == ENUM_HVBPRESTA_PRECOOL]
        | {VPMM_PwrStaConstraint_enum = ENUM_PWRCONSTRAINT_HVACTIVE;}
    (junction 7) -> (junction 80) [order 2]
    (junction 8) -> (junction 9) : {VPMM_TCountSta_enum = ENUM_TCOUNTSTA_NOCOUNTING;
        |  VPMM_PwrOffTimer_s = 0;
        |  VPMM_ConstraintLoop_flg = TRUE;}
    (junction 80) -> (junction 82) [order 1] : [VPMM_TCountSta_enum == ENUM_TCOUNTSTA_COUNTINGFINISH]
    (junction 82) -> (junction 90) [order 1] : [VPMM_PwrStaSW_enum == ENUM_PWRSTASW_PWRDOWN]
    (junction 80) -> (junction 10) [order 2]
    (junction 82) -> (junction 84) [order 2]
    (junction 90) -> (junction 92) : {VPMM_TCountSta_enum = ENUM_TCOUNTSTA_NOCOUNTING;}
    (junction 10) -> (junction 11) [order 1] : [(VPMM_PowerOffTSet_s > 0 && ...
        |   (VINP_RePwrReqTbox_enum == ENUM_REPWRREQTBOX_REQVEHCHK || ...
        |    VINP_RePwrReqTbox_enum == ENUM_REPWRREQTBOX_REQDTC || ...
        |    VINP_RePwrReqTbox_enum == ENUM_REPWRREQTBOX_REQRADIO || ...
        |    VINP_RePwrReqTbox_enum == ENUM_REPWRREQTBOX_REQON)) || ...
        |  (VPMM_PowerOffTSetDKC_enum > 0 && ...
        |   (VINP_RePwrReqDKCT_enum == ENUM_REPWRREQDKC_REQVEHCHK || ...
        |    VINP_RePwrReqDKCT_enum == ENUM_REPWRREQDKC_REQDTC || ...
        |    VINP_RePwrReqDKCT_enum == ENUM_REPWRREQDKC_REQRADIO || ...
        |    VINP_RePwrReqDKCT_enum == ENUM_REPWRREQDKC_REQON))]
    (junction 10) -> (junction 12) [order 2]
    (junction 11) -> (junction 13) : {VPMM_PwrStaConstraint_enum = ENUM_PWRCONSTRAINT_ONFORTIME;}
    (junction 12) -> (junction 13) [order 1] : [(VPMM_PowerOffTSet_s > 0 && ...
        |   VINP_RePwrReqTbox_enum == ENUM_REPWRREQTBOX_REQACTEMP) || ...
        |  (VPMM_PowerOffTSetDKC_enum > 0 && ...
        |   VINP_RePwrReqDKCT_enum == ENUM_REPWRREQDKC_REQACTEMP)]
        | {VPMM_PwrStaConstraint_enum = ENUM_PWRCONSTRAINT_HVFORTIME;}
    (junction 13) -> (junction 14) [order 1] : [(VPMM_PowerOffTSet_s >= VPMM_PowerOffTSetDKC_enum && VPMM_PwrOffTimer_s >= VPMM_PowerOffTSet_s) || ...
        |  (VPMM_PowerOffTSetDKC_enum > VPMM_PowerOffTSet_s && VPMM_PwrOffTimer_s >= VPMM_PowerOffTSetDKC_enum)]
    (junction 12) -> (junction 15) [order 2] : {VPMM_TCountSta_enum = ENUM_TCOUNTSTA_NOCOUNTING;
        |  VPMM_PwrOffTimer_s = 0;}
    (junction 13) -> (junction 16) [order 2] : {VPMM_TCountSta_enum = ENUM_TCOUNTSTA_TIMMERCOUNTING;
        |  VPMM_PwrOffTimer_s += task_time_s;
        |  VPMM_ConstraintLoop_flg = TRUE;}
    (junction 14) -> (junction 17) : {VPMM_TCountSta_enum = ENUM_TCOUNTSTA_COUNTINGFINISH;
        |  VPMM_PwrStaConstraint_enum = ENUM_PWRCONSTRAINT_NOREQUEST;
        |  VPMM_PwrOffTimer_s = 0;}
  data: task_time_s input; VPMM_PowerSta_enum input; VINP_AVMOFFRecButt_flg input; VINP_HVBPreheatPrecoolSta_enum input; VINP_OFFACMODE_enum input; VPMM_PowerOffTSet_s input; VPMM_PowerOffTSetDKC_enum input; VINP_PwrReq_OTA_enum input; VINP_RePwrReqDKCT_enum input; VINP_RePwrReqTbox_enum input; VPMM_PwrStaConstraint_enum output; VPMM_TCountSta_enum output; VPMM_PwrOffTimer_s local single; ENUM_AVMOFFRECBUTT_ON parameter; ENUM_HVBPRESTA_PRECOOL parameter; ENUM_HVBPRESTA_PREHEAT parameter; ENUM_OFFACMODE_CAMP parameter; ENUM_OFFACMODE_ON parameter; ENUM_OFFACMODE_PET parameter; ENUM_POWERSTA_OFFA parameter; ENUM_POWERSTA_OFFC parameter; ENUM_POWERSTA_ON parameter; ENUM_PWRCONSTRAINT_HVACTIVE parameter; ENUM_PWRCONSTRAINT_HVFORTIME parameter; ENUM_PWRCONSTRAINT_NOREQUEST parameter; ENUM_PWRCONSTRAINT_ONFORTIME parameter; ENUM_PWRCONSTRAINT_PWRSTAON parameter; ENUM_PWRREQOTA_REQPOWERON parameter; ENUM_REPWRREQDKC_REQACTEMP parameter; ENUM_REPWRREQDKC_REQDTC parameter; ENUM_REPWRREQDKC_REQON parameter; ENUM_REPWRREQDKC_REQRADIO parameter; ENUM_REPWRREQDKC_REQVEHCHK parameter; ENUM_REPWRREQTBOX_REQACTEMP parameter; ENUM_REPWRREQTBOX_REQDTC parameter; ENUM_REPWRREQTBOX_REQON parameter; ENUM_REPWRREQTBOX_REQRADIO parameter; ENUM_REPWRREQTBOX_REQVEHCHK parameter; ENUM_TCOUNTSTA_COUNTINGFINISH parameter; ENUM_TCOUNTSTA_NOCOUNTING parameter; ENUM_TCOUNTSTA_TIMMERCOUNTING parameter; VPMM_ConstraintLoop_flg local boolean; FALSE parameter; TRUE parameter; VPMM_PwrStaSW_enum input; ENUM_PWRSTASW_PWRDOWN parameter
